simulink model "sf_test"  (R2020a)
settings: Solver=FixedStepDiscrete  StartTime=0.0  StopTime=10.0  RelTol=1e-3
settings Model: Creator=김진성  LastModifiedBy=김진성
settings OptimizationCC: DefaultParameterBehavior=Inlined  EnhancedBackFolding=on  PassReuseOutputArgsAs=Individual arguments  OptimizeBlockOrder=speed  DifferentSizesBufferReuse=on  OptimizationCustomize=off  EfficientTunableParamExpr=on
settings DebuggingCC: ParameterTunabilityLossMsg=error
settings HardwareCC: ProdBitPerPointer=32  ProdBitPerSizeT=32  ProdBitPerPtrDiffT=32  ProdLargestAtomicInteger=Long  ProdLargestAtomicFloat=Double  ProdWordSize=32  ProdHWDeviceType=ARM Compatible->ARM Cortex
settings SFSimCC: MATLABDynamicMemAlloc=off
settings RTWCC: SystemTargetFile=ert.tlc  GenCodeOnly=on  TemplateMakefile=ert_default_tmf  GenerateReport=on  IncludeHyperlinkInReport=on  LaunchReport=on  GenerateTraceInfo=on  GenerateTraceReport=on  GenerateTraceReportSl=on  GenerateTraceReportSf=on  GenerateTraceReportEml=on  GenerateCodeMetricsReport=on  GenerateCodeReplacementReport=on
settings CodeAppCC: ForceParamTrailComments=on  IgnoreCustomStorageClasses=off  OperatorAnnotations=on  SimulinkDataObjDesc=on  SFDataObjDesc=on  InsertBlockDesc=on  StateflowObjectComments=on
settings ERTTargetCC: TargetLangStandard=C99 (ISO)  GenerateSampleERTMain=on  MultiInstanceERTCode=on  CodeInterfacePackaging=Reusable function  InlinedParameterPlacement=NonHierarchical  ERTCustomFileTemplate=example_file_process.tlc

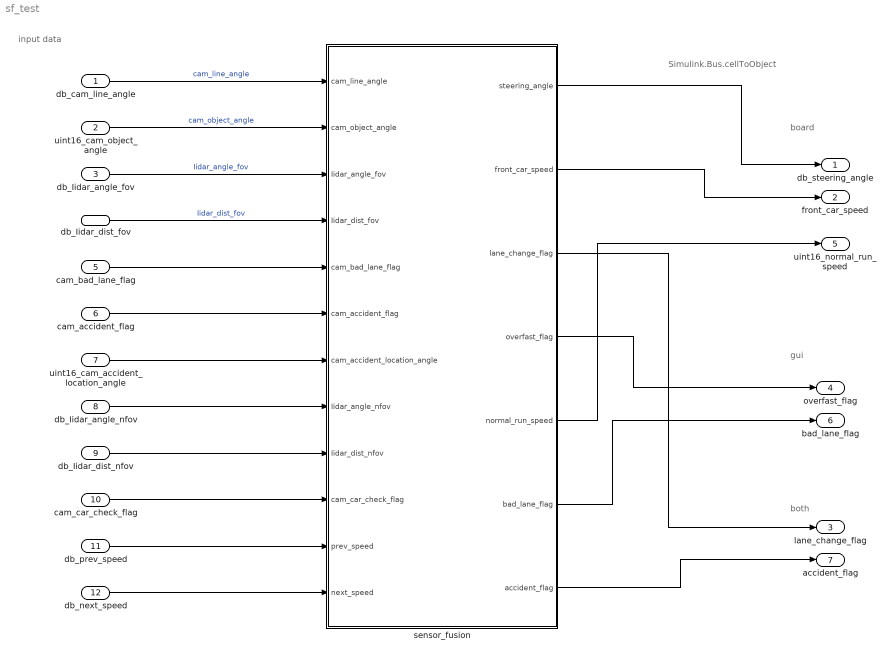
== system sf_test ==
  note: Simulink.Bus.cellToObject
  note: both
  note: gui
  note: board
  note: input data
  db_cam_line_angle : Inport
  uint16_cam_object_angle : Inport  Port=2  OutDataTypeStr=uint16
  db_Iidar_angle_fov : Inport  Port=3
  db_Iidar_dist_fov : Inport  Port=4
  cam_bad_lane_flag : Inport  Port=5  OutDataTypeStr=boolean
  cam_accident_flag : Inport  Port=6  OutDataTypeStr=boolean
  uint16_cam_accident_location_angle : Inport  Port=7  OutDataTypeStr=uint16
  db_Iidar_angle_nfov : Inport  Port=8
  db_Iidar_dist_nfov : Inport  Port=9
  cam_car_check_flag : Inport  Port=10  OutDataTypeStr=boolean
  db_prev_speed : Inport  Port=11
  db_next_speed : Inport  Port=12
  sensor_fusion : Subsystem  TreatAsAtomicUnit=on
      settings: RTWSystemCode=Nonreusable function  RTWFcnNameOpts=Use subsystem name
  db_steering_angle : Outport
  front_car_speed : Outport  Port=2
  lane_change_flag : Outport  Port=3
  overfast_flag : Outport  Port=4
  uint16_normal_run_speed : Outport  Port=5  OutDataTypeStr=uint16
  bad_lane_flag : Outport  Port=6
  accident_flag : Outport  Port=7
  wires:
  db_Iidar_angle_fov/1 -> sensor_fusion/3(Iidar_angle_fov)  "Iidar_angle_fov"
  cam_accident_flag/1 -> sensor_fusion/6(cam_accident_flag)
  db_Iidar_dist_fov/1 -> sensor_fusion/4(Iidar_dist_fov)  "Iidar_dist_fov"
  db_Iidar_angle_nfov/1 -> sensor_fusion/8(Iidar_angle_nfov)
  db_cam_line_angle/1 -> sensor_fusion/1(cam_line_angle)  "cam_line_angle"
  db_Iidar_dist_nfov/1 -> sensor_fusion/9(Iidar_dist_nfov)
  cam_car_check_flag/1 -> sensor_fusion/10(cam_car_check_flag)
  cam_bad_lane_flag/1 -> sensor_fusion/5(cam_bad_lane_flag)
  uint16_cam_object_angle/1 -> sensor_fusion/2(cam_object_angle)  "cam_object_angle"
  uint16_cam_accident_location_angle/1 -> sensor_fusion/7(cam_accident_location_angle)
  sensor_fusion/1(steering_angle) -> db_steering_angle/1
  db_prev_speed/1 -> sensor_fusion/11(prev_speed)
  db_next_speed/1 -> sensor_fusion/12(next_speed)
  sensor_fusion/3(lane_change_flag) -> lane_change_flag/1
  sensor_fusion/4(overfast_flag) -> overfast_flag/1
  sensor_fusion/5(normal_run_speed) -> uint16_normal_run_speed/1
  sensor_fusion/2(front_car_speed) -> front_car_speed/1
  sensor_fusion/6(bad_lane_flag) -> bad_lane_flag/1
  sensor_fusion/7(accident_flag) -> accident_flag/1

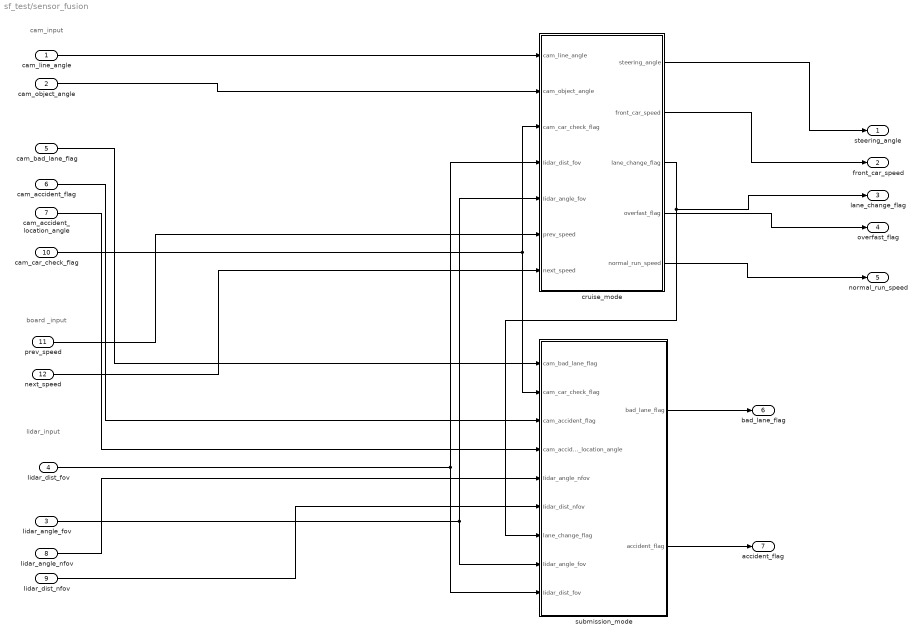
== system sf_test/sensor_fusion ==
  note: board _input
  note: lidar_input
  note: cam_input
  cam_line_angle : Inport
  cam_object_angle : Inport  Port=2
  Iidar_angle_fov : Inport  Port=3
  Iidar_dist_fov : Inport  Port=4
  cam_bad_lane_flag : Inport  Port=5
  cam_accident_flag : Inport  Port=6
  cam_accident_location_angle : Inport  Port=7
  Iidar_angle_nfov : Inport  Port=8
  Iidar_dist_nfov : Inport  Port=9
  cam_car_check_flag : Inport  Port=10
  prev_speed : Inport  Port=11
  next_speed : Inport  Port=12
  cruise_mode : Subsystem  TreatAsAtomicUnit=on
      settings: RTWSystemCode=Nonreusable function  RTWFcnNameOpts=Use subsystem name
  submission_mode : Subsystem  TreatAsAtomicUnit=on
      settings: RTWSystemCode=Nonreusable function  RTWFcnNameOpts=Use subsystem name
  steering_angle : Outport
  front_car_speed : Outport  Port=2
  lane_change_flag : Outport  Port=3
  overfast_flag : Outport  Port=4
  normal_run_speed : Outport  Port=5  OutDataTypeStr=uint16
  bad_lane_flag : Outport  Port=6
  accident_flag : Outport  Port=7
  wires:
  cam_line_angle/1 -> cruise_mode/1(cam_line_angle)
  cam_object_angle/1 -> cruise_mode/2(cam_object_angle)
  cam_accident_flag/1 -> submission_mode/3(cam_accident_flag)
  cam_accident_location_angle/1 -> submission_mode/4(cam_accident_location_angle)
  Iidar_angle_nfov/1 -> submission_mode/5(Iidar_angle_nfov)
  Iidar_dist_nfov/1 -> submission_mode/6(Iidar_dist_nfov)
  cam_bad_lane_flag/1 -> submission_mode/1(cam_bad_lane_flag)
  cam_car_check_flag/1 -> submission_mode/2(cam_car_check_flag), cruise_mode/3(cam_car_check_flag)
  cruise_mode/1(steering_angle) -> steering_angle/1
  prev_speed/1 -> cruise_mode/6(prev_speed)
  next_speed/1 -> cruise_mode/7(next_speed)
  cruise_mode/2(front_car_speed) -> front_car_speed/1
  cruise_mode/4(overfast_flag) -> overfast_flag/1
  cruise_mode/3(lane_change_flag) -> submission_mode/7(lane_change_flag), lane_change_flag/1
  cruise_mode/5(normal_run_speed) -> normal_run_speed/1
  Iidar_angle_fov/1 -> cruise_mode/5(Iidar_angle_fov), submission_mode/8(Iidar_angle_fov)
  Iidar_dist_fov/1 -> submission_mode/9(Iidar_dist_fov), cruise_mode/4(Iidar_dist_fov)
  submission_mode/1(bad_lane_flag) -> bad_lane_flag/1
  submission_mode/2(accident_flag) -> accident_flag/1

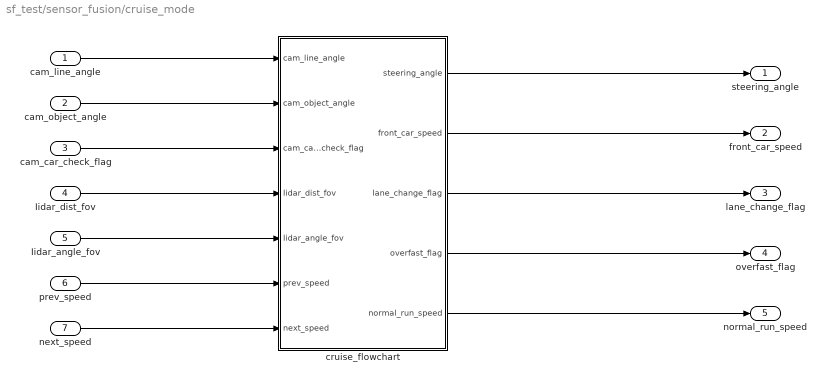
== system sf_test/sensor_fusion/cruise_mode ==
  cam_line_angle : Inport
  cam_object_angle : Inport  Port=2
  cam_car_check_flag : Inport  Port=3
  Iidar_dist_fov : Inport  Port=4
  Iidar_angle_fov : Inport  Port=5
  prev_speed : Inport  Port=6
  next_speed : Inport  Port=7
  cruise_flowchart : Stateflow chart  TreatAsAtomicUnit=on
      settings: RTWSystemCode=Nonreusable function  RTWFcnNameOpts=Use subsystem name
  steering_angle : Outport
  front_car_speed : Outport  Port=2
  lane_change_flag : Outport  Port=3
  overfast_flag : Outport  Port=4
  normal_run_speed : Outport  Port=5  OutDataTypeStr=uint16
  wires:
  cam_line_angle/1 -> cruise_flowchart/1(cam_line_angle)
  cam_object_angle/1 -> cruise_flowchart/2(cam_object_angle)
  cam_car_check_flag/1 -> cruise_flowchart/3(cam_car_check_flag)
  Iidar_dist_fov/1 -> cruise_flowchart/4(Iidar_dist_fov)
  Iidar_angle_fov/1 -> cruise_flowchart/5(Iidar_angle_fov)
  cruise_flowchart/1(steering_angle) -> steering_angle/1
  cruise_flowchart/2(front_car_speed) -> front_car_speed/1
  prev_speed/1 -> cruise_flowchart/6(prev_speed)
  next_speed/1 -> cruise_flowchart/7(next_speed)
  cruise_flowchart/3(lane_change_flag) -> lane_change_flag/1
  cruise_flowchart/4(overfast_flag) -> overfast_flag/1
  cruise_flowchart/5(normal_run_speed) -> normal_run_speed/1

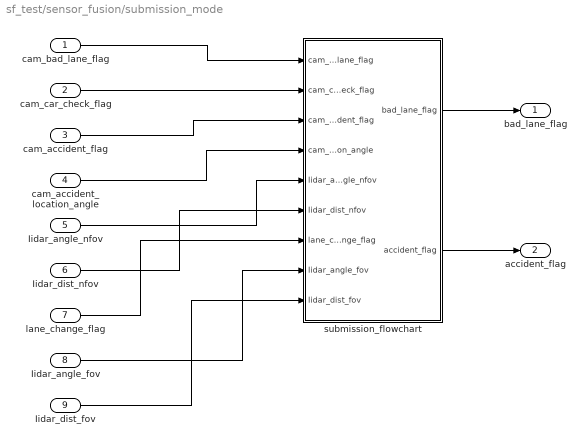
== system sf_test/sensor_fusion/submission_mode ==
  cam_bad_lane_flag : Inport
  cam_car_check_flag : Inport  Port=2
  cam_accident_flag : Inport  Port=3
  cam_accident_location_angle : Inport  Port=4
  Iidar_angle_nfov : Inport  Port=5
  Iidar_dist_nfov : Inport  Port=6
  lane_change_flag : Inport  Port=7
  Iidar_angle_fov : Inport  Port=8
  Iidar_dist_fov : Inport  Port=9
  submission_flowchart : Stateflow chart  TreatAsAtomicUnit=on
      settings: RTWSystemCode=Nonreusable function  RTWFcnNameOpts=Use subsystem name
  bad_lane_flag : Outport
  accident_flag : Outport  Port=2
  wires:
  cam_bad_lane_flag/1 -> submission_flowchart/1(cam_bad_lane_flag)
  cam_car_check_flag/1 -> submission_flowchart/2(cam_car_check_flag)
  cam_accident_flag/1 -> submission_flowchart/3(cam_accident_flag)
  cam_accident_location_angle/1 -> submission_flowchart/4(cam_accident_location_angle)
  Iidar_angle_nfov/1 -> submission_flowchart/5(Iidar_angle_nfov)
  Iidar_dist_nfov/1 -> submission_flowchart/6(Iidar_dist_nfov)
  lane_change_flag/1 -> submission_flowchart/7(lane_change_flag)
  Iidar_angle_fov/1 -> submission_flowchart/8(Iidar_angle_fov)
  Iidar_dist_fov/1 -> submission_flowchart/9(Iidar_dist_fov)
  submission_flowchart/1(bad_lane_flag) -> bad_lane_flag/1
  submission_flowchart/2(accident_flag) -> accident_flag/1

== stateflow chart sf_test/sensor_fusion/submission_mode/submission_flowchart ==
  state init_func
    state init
    state local_variable_init
      entry:
      local_lidar_dist_nfov = Iidar_dist_nfov;
      local_lider_angle_nfov = Iidar_angle_nfov;
      local_lidar_angle_fov = Iidar_angle_fov;
      local_lidar_dist_fov = Iidar_dist_fov;
    (default) -> init
    init -> local_variable_init [order 1] : [cam_car_check_flag==1]
  state bad_lane_func
    entry:
    bad_lane_flag = 1;
  note: -input data -
      | cam_bad_lane_flag
      | cam_car_check_flag
      | cam_accident_flag
      |
      | cam_accident_location_angle
      |
      | Iidar_angle_nfov
      | Iidar_dist_nfov
      | Iidar_angle_fov
      | Iidar_dist_fov
      |
      | lane_change_flag
  note: -output data -
      |
      | bad_lane_flag
      | accident_flag
  state accident_func
    entry:
    local_accident_location_angle = cam_accident_location_angle;
    accident_flag = 1;
  state lane_change_func
    entry:
  note: locla_variable_init 내부에 로컬 라이다 데이터(fov,nfov) 관련 처리 흐름도 추가할 것
  (default) -> init_func
  init -> bad_lane_func [order 2] : [cam_bad_lane_flag==1]
  local_variable_init -> accident_func [order 1] : [cam_accident_flag==1]
  local_variable_init -> lane_change_func [order 2] : [lane_change_flag==1]
  data: cam_bad_lane_flag input; cam_car_check_flag input; cam_accident_flag input; cam_accident_location_angle input; Iidar_angle_nfov input; Iidar_dist_nfov input; lane_change_flag input; local_lidar_dist_nfov local; local_lider_angle_nfov local; local_accident_location_angle local; Iidar_angle_fov input; Iidar_dist_fov input; local_lidar_angle_fov local; local_lidar_dist_fov local; bad_lane_flag output; accident_flag output

== stateflow chart sf_test/sensor_fusion/cruise_mode/cruise_flowchart ==
  state front_car_decision
    state decision_init
      entry:
      local_object_angle = cam_object_angle;
      local_line_angle = cam_line_angle;
      local_current_speed_avr = ( ( prev_speed + next_speed ) /2 );
      exit :
      disp("decision_init_exit");
    state calculate_speed_logic
      entry:
      steering_angle = local_line_angle;
      local_dist_diff = 0;
    state fast_speed_state
      entry:
      overfast_flag = 1;
    state low_speed_state
      entry:
      lane_change_flag = 1;
    (default) -> decision_init
    decision_init -> calculate_speed_logic
    calculate_speed_logic -> fast_speed_state [order 1] : [front_car_speed > local_current_speed_avr]
    calculate_speed_logic -> low_speed_state [order 2] : [front_car_speed < local_current_speed_avr]
  state normal_run
    %normal run func
    entry:
    steering_angle = cam_line_angle;
    front_car_speed = 0;
    car_check = 1;
    exit:
    normal_run_speed = 1000;
    disp("normal_run exit");
  note: - input data -
      |
      | cam_line_angle
      | cam_object_angle
      | cam_car_check_flag
      | cam_bad_lane_flag
      | cam_accident_flag
      | cam_accident_location_angle
      |
      | lidar_dist_fov
      | lidar_angle_fov
      |
      | lidar_dist_nfov
      | lidar_angle_nfov
      |
      | prev_speed
      | next_speed
  note: - output data -
      |
      | steering_angle
      | front_car_speed
      | lane_change_flag
      | normal_run_speed
  (default) -> normal_run
  normal_run -> front_car_decision [order 1] : [cam_car_check_flag == 1]
  normal_run -> front_car_decision [order 2] : [car_check==1]
  data: cam_line_angle input; cam_object_angle input; cam_car_check_flag input; Iidar_dist_fov input; Iidar_angle_fov input; steering_angle output; local_object_angle local; local_line_angle local; local_current_speed_avr local; front_car_speed output; local_dist_diff local; prev_speed input; next_speed input; lane_change_flag output; overfast_flag output; car_check local double; normal_run_speed output uint16
